simulink model "Zaeher"  (R2021a)
settings: Solver=ode3  StartTime=0.0  StopTime=10.0  FixedStep=0.01  RelTol=1e-3
libraries: simulink x1
settings Model: Creator=Oceaner  LastModifiedBy=Oceaner

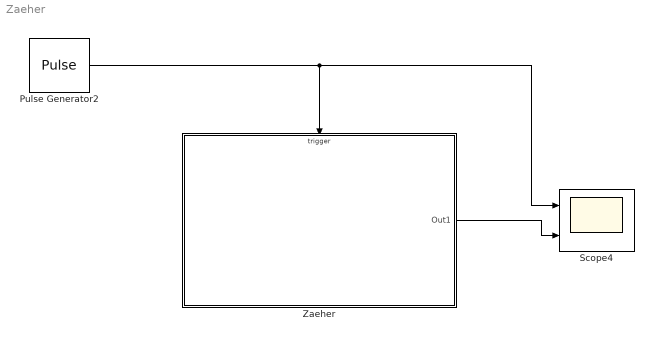
== system Zaeher ==
  " Zaeher" : Subsystem  TreatAsAtomicUnit=on
  Pulse Generator2 : DiscretePulseGenerator  PulseType=Time based  PulseWidth=50
  Scope4 : Scope  NumInputPorts=2
  wires:
  " Zaeher"/1(Out1) -> Scope4/2
  Pulse Generator2/1 -> Scope4/1, " Zaeher"/Trigger

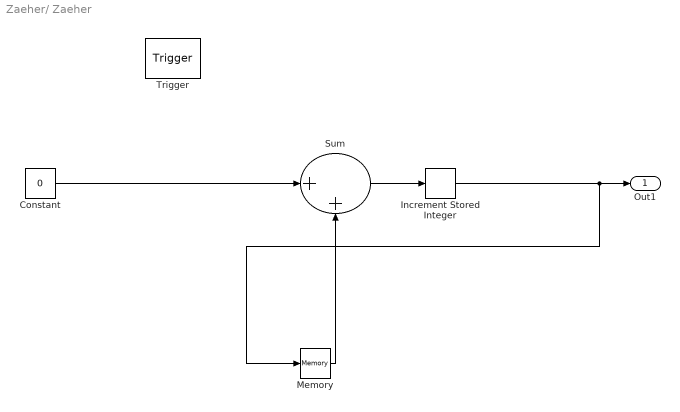
== system Zaeher/ Zaeher ==
  Trigger : TriggerPort  VariantControl=(inherit)
  Constant : Constant  Value=0
  Increment Stored Integer : simulink/Additional Math & Discrete/Additional Math: Increment - Decrement/Increment Stored Integer
  Memory : Memory  InheritSampleTime=on
  Sum : Sum  Inputs=|++
  Out1 : Outport
  wires:
  Sum/1 -> Increment Stored Integer/1
  Memory/1 -> Sum/2
  Constant/1 -> Sum/1
  Increment Stored Integer/1 -> Out1/1, Memory/1
